simulink model "Highpass_filter"  (R2020b)
settings: Solver=VariableStepAuto  StartTime=0.0  StopTime=10.0  RelTol=1e-3
settings Model: Creator=shubham sharma  LastModifiedBy=shubham sharma

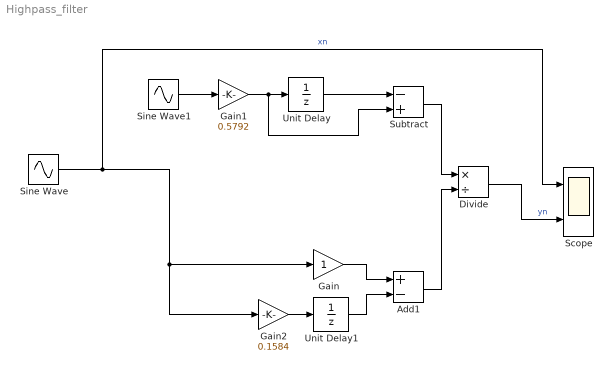
== system Highpass_filter ==
  Add1 : Sum  Inputs=+-
  Divide : Product  Inputs=*/
  Gain : Gain
  Gain1 : Gain  Gain=0.5792
  Gain2 : Gain  Gain=0.1584
  Scope : Scope  NumInputPorts=2
  Sine Wave : Sin  Frequency=310  SampleTime=0
  Sine Wave1 : Sin  SampleTime=0
  Subtract : Sum  Inputs=-+
  Unit Delay : UnitDelay  SampleTime=-1  HasFrameUpgradeWarning=on
  Unit Delay1 : UnitDelay  SampleTime=-1  HasFrameUpgradeWarning=on
  wires:
  Subtract/1 -> Divide/1
  Gain/1 -> Add1/1
  Gain2/1 -> Unit Delay1/1
  Unit Delay1/1 -> Add1/2
  Add1/1 -> Divide/2
  Sine Wave/1 -> Scope/1, Gain2/1, Gain/1  "xn"
  Divide/1 -> Scope/2  "yn"
  Gain1/1 -> Unit Delay/1, Subtract/2
  Unit Delay/1 -> Subtract/1
  Sine Wave1/1 -> Gain1/1
